simulink model "ThreePhaseVolSourceInv"  (R2017b)
settings: Solver=VariableStepAuto  StartTime=0.0  StopTime=2  MaxStep=1e-4  RelTol=1e-3
libraries: powerlib x16
settings Model: Creator=india  LastModifiedBy=india

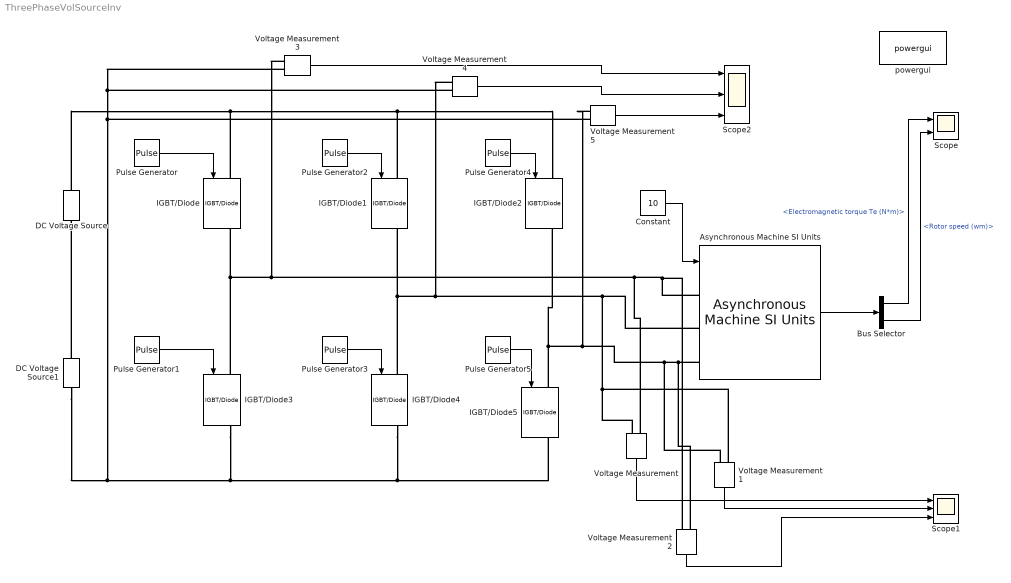
== system ThreePhaseVolSourceInv ==
  Asynchronous Machine SI Units : powerlib/Machines/Asynchronous Machine SI Units  RotorType=Squirrel-cage  PresetModel="15:  5.4 HP (4KW)   400 V  50Hz 1430 RPM"  MechanicalLoad=Torque Tm  ShowDetailedParameters=on  ReferenceFrame=Rotor  Units=SI  MeasurementBus=off  NominalParameters=[4000 400 50]  Stator=[1.405 0.005839]  Rotor=[1.395 0.005839]  Cage1=[0.4155 0.002066]  Cage2=[0.4168 0.0003495]  Lm=0.1722  Mechanical=[0.0131 0.002985 2]  PolePairs=2  InitialConditions=[0 0 0 0 0 0 0 0]  SimulateSaturation=off  Saturation=[14.03593122, 27.81365428, 53.79336849, 72.68890987, 97.98006896, 148.6815601, 215.7428561, 302.9841135, 428.7778367 ; 230, 322, 414, 460, 506, 552, 598, 644, 690]  LoadFlowParameters=1492000  TsPowergui=0  TsBlock=-1  IterativeModel=Trapezoidal non iterative  IterativeDiscreteModel=Trapezoidal non iterative  Pmec=1.492e+006
  Bus Selector : BusSelector  OutputSignals=Mechanical.Electromagnetic torque Te (N*m),Mechanical.Rotor speed (wm)
  Constant : Constant  Value=10
  DC Voltage Source : powerlib/Electrical Sources/DC Voltage Source  Amplitude=200*sqrt(2)  Measurements=None
  DC Voltage Source1 : powerlib/Electrical Sources/DC Voltage Source  Amplitude=200 * sqrt(2)  Measurements=None
  IGBT/Diode{,1..5} (6 alike) : powerlib/Power Electronics/IGBT//Diode  Ron=1e-3  Rs=1e5  Cs=inf  Measurements=on
  Pulse Generator : DiscretePulseGenerator  PulseType=Time based  Period=20e-03  PulseWidth=50  PhaseDelay=3.33e-03
  Pulse Generator1 : DiscretePulseGenerator  PulseType=Time based  Period=20e-03  PulseWidth=50  PhaseDelay=13.33e-03
  Pulse Generator2 : DiscretePulseGenerator  PulseType=Time based  Period=20e-03  PulseWidth=50  PhaseDelay=10e-03
  Pulse Generator3 : DiscretePulseGenerator  PulseType=Time based  Period=20e-03  PulseWidth=50  PhaseDelay=20e-03
  Pulse Generator4 : DiscretePulseGenerator  PulseType=Time based  Period=20e-03  PulseWidth=50  PhaseDelay=16.66e-03
  Pulse Generator5 : DiscretePulseGenerator  PulseType=Time based  Period=20e-03  PulseWidth=50  PhaseDelay=6.66e-03
  Scope : Scope  NumInputPorts=2
  Scope1 : Scope  NumInputPorts=3
  Scope2 : Scope  NumInputPorts=3
  Voltage Measurement{,1..5} (6 alike) : powerlib/Measurements/Voltage Measurement  PhasorSimulation=off  OutputType=Complex  PSBequivalent=0
  powergui : powerlib/powergui  Priority=1  SimulationMode=Continuous  SampleTime=50e-6  frequency=60  Iterations=50  frequencyindice=50  Pbase=100e6  ErrMax=1e-4  UnitsV=kV  UnitsW=MW  buscounter=0  FunctionMessages=off  echomessages=off  EnableUseOfTLC=off  CurrentSourceSwitches=off  DisableSnubberDevices=off  DisableRonSwitches=off  DisableVfSwitches=off  DisplayEquations=off  SolverType=Tustin/Backward Euler (TBE)  Interpol=off  ExternalGateDelay=off  methode=off  Ts=100  x0status=blocks  SPID=on  SwTol=0  HookPort=off  RestoreLinks=warning  ResistiveCurrentMeasurement=off  Frange=[0:2:500]  Ylog=off  Xlog=on  ShowGrid=off  save=off  variable=ZData  structure=0  ZoomFFT=off  StartTime=0.0  cycles=1  DisplayStyle=1  fundamental=60  FreqAxis=off  MaxFrequency=1000  frequencyindicesteady=1  RmsSteady=1  display=off
  wires:
  Pulse Generator4/1 -> IGBT/Diode2/1
  Pulse Generator5/1 -> IGBT/Diode5/1
  Pulse Generator2/1 -> IGBT/Diode1/1
  Pulse Generator3/1 -> IGBT/Diode4/1
  Pulse Generator/1 -> IGBT/Diode/1
  Pulse Generator1/1 -> IGBT/Diode3/1
  Constant/1 -> Asynchronous Machine SI Units/1
  Asynchronous Machine SI Units/1 -> Bus Selector/1
  Bus Selector/1 -> Scope/1  "<Electromagnetic torque Te (N*m)>"
  Bus Selector/2 -> Scope/2  "<Rotor speed (wm)>"
  Voltage Measurement/1 -> Scope1/1
  Voltage Measurement1/1 -> Scope1/2
  Voltage Measurement2/1 -> Scope1/3
  Voltage Measurement3/1 -> Scope2/1
  Voltage Measurement4/1 -> Scope2/2
  Voltage Measurement5/1 -> Scope2/3
  connections:
  DC Voltage Source1/RConn1 -- DC Voltage Source/LConn1
  DC Voltage Source1/LConn1 -- Voltage Measurement5/LConn2 -- Voltage Measurement4/LConn2 -- Voltage Measurement3/LConn2 -- IGBT/Diode3/RConn1 -- IGBT/Diode4/RConn1 -- IGBT/Diode5/RConn1
  DC Voltage Source/RConn1 -- IGBT/Diode/LConn1 -- IGBT/Diode1/LConn1 -- IGBT/Diode2/LConn1
  IGBT/Diode3/LConn1 -- Voltage Measurement3/LConn1 -- Voltage Measurement2/LConn2 -- Asynchronous Machine SI Units/LConn1 -- Voltage Measurement/LConn1 -- IGBT/Diode/RConn1
  IGBT/Diode4/LConn1 -- Voltage Measurement4/LConn1 -- Voltage Measurement1/LConn1 -- Voltage Measurement/LConn2 -- Asynchronous Machine SI Units/LConn2 -- IGBT/Diode1/RConn1
  IGBT/Diode5/LConn1 -- Voltage Measurement5/LConn1 -- Voltage Measurement2/LConn1 -- Asynchronous Machine SI Units/LConn3 -- Voltage Measurement1/LConn2 -- IGBT/Diode2/RConn1
